simulink model "bikeBBR_gesloopt"  (Simulink 7.4)
settings: Solver=ode23s  StartTime=0.0  StopTime=50  RelTol=1e-3
values from neighbouring files (symbols this model uses):
  ABBR = [0 8.39044421109 0 8.09876894767 1 -0.112133410006 0 6.81426106958 0 -17.7563110842 0 -7.30629683726 ... (16 elements, 4x4)]    [BBR.mat]
  BBBR = [0  0; 0.0105572020466  -0.0498370711137; 0  0; -0.0498370711137  3.02856047537]    [BBR.mat]
  CBBR = [1 0 0 0 0 1 0 0 0 0 1 0 ... (16 elements, 4x4)]    [BBR.mat]
  DBBR = [0  0; 0  0; 0  0; 0  0]    [BBR.mat]
  kagress = 1    [BBR.mat]
  Kdelta = X(3)    [H_bikeplusrider.m]
  Kphi = X(1)    [H_bikeplusrider.m]
  Kphid = X(2)    [H_bikeplusrider.m]
libraries: simulink x1
settings Model: Creator=Peter  LastModifiedBy=Peter
settings OptimizationCC: InlineParams=on  InlineInvariantSignals=on  InitFltsAndDblsToZero=on
settings DebuggingCC: SaveWithParameterizedLinksMsg=none  SignalResolutionControl=TryResolveAllWithWarning  MultiTaskDSMMsg=warning  MultiTaskCondExecSysMsg=none  StrictBusMsg=None
settings RTWCC: IncludeERTFirstTime=on
settings GRTTargetCC: TargetFcnLib=ansi_tfl_tmw.mat

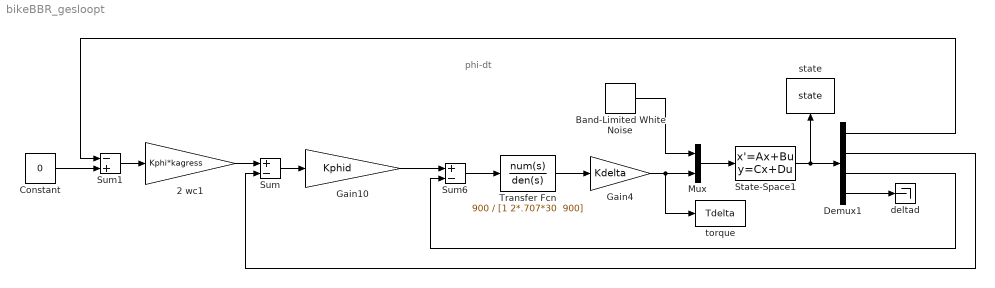
== system bikeBBR_gesloopt ==
  note: phi-dt
  2 wc1 : Gain  Gain=Kphi*kagress  ParameterDataType=sfix(16)  ParameterScaling=2^0  OutDataType=sfix(16)  OutScaling=2^0
  Band-Limited White Noise : simulink/Sources/Band-Limited White Noise  SystemSampleTime=-1  Cov=[0.1]  Ts=0.1  seed=[23341]
  Constant : Constant  Value=0  OutDataType=fixdt(1, 16)  OutScaling=2^0
  Demux1 : Demux
  Gain10 : Gain  Gain=Kphid  ParameterDataType=sfix(16)  ParameterScaling=2^0  OutDataType=sfix(16)  OutScaling=2^0
  Gain4 : Gain  Gain=Kdelta  ParameterDataType=sfix(16)  ParameterScaling=2^0  OutDataType=sfix(16)  OutScaling=2^0
  Mux : Mux  Inputs=2
  State-Space1 : StateSpace  A=ABBR  B=BBBR  C=CBBR  D=DBBR
  Sum : Sum  Inputs=+-  OutDataType=sfix(16)  OutScaling=2^0
  Sum1 : Sum  Inputs=-+  OutDataType=sfix(16)  OutScaling=2^0
  Sum6 : Sum  Inputs=+-  OutDataType=sfix(16)  OutScaling=2^0
  Transfer Fcn : TransferFcn  Numerator=900  Denominator="[1 2*.707*30  900]"
  deltad : Terminator
  state : ToWorkspace  VariableName=state  SampleTime=-1  SaveFormat=Array
  torque : ToWorkspace  VariableName=Tdelta  SampleTime=-1  SaveFormat=Array
  wires:
  Sum/1 -> Gain10/1
  State-Space1/1 -> Demux1/1, state/1
  Demux1/2 -> Sum/2
  Transfer Fcn/1 -> Gain4/1
  Sum6/1 -> Transfer Fcn/1
  Sum1/1 -> 2 wc1/1
  Demux1/1 -> Sum1/1
  Gain10/1 -> Sum6/1
  Demux1/3 -> Sum6/2
  2 wc1/1 -> Sum/1
  Demux1/4 -> deltad/1
  Constant/1 -> Sum1/2
  Mux/1 -> State-Space1/1
  Gain4/1 -> Mux/2, torque/1
  Band-Limited White Noise/1 -> Mux/1
